simulink model "FieLew95_r2018a"  (R2018a)
settings: Solver=ode1  StartTime=0.0  StopTime=10  FixedStep=0.01  RelTol=1e-5  EnableMultiTasking=on
libraries: simulink x1
settings Model: Creator=dwbertol  LastModifiedBy=dwbertol
settings DataIOCC: LimitDataPoints=on  SaveFormat=Array  SignalLoggingSaveFormat=ModelDataLogs
settings OptimizationCC: ExpressionDepthLimit=2147483647  LifeSpan=inf
settings DebuggingCC: UnderspecifiedInitializationDetection=Classic  MergeDetectMultiDrivingBlocksExec=none  SolverPrmCheckMsg=warning  FcnCallInpInsideContextMsg=warning  StateNameClashWarn=warning  SFUnexpectedBacktrackingDiag=warning  SFNoUnconditionalDefaultTransitionDiag=warning  SFExecutionAtInitializationDiag=none
settings HardwareCC: ProdBitPerPointer=32  ProdBitPerSizeT=32  ProdBitPerPtrDiffT=32  ProdLargestAtomicFloat=None  ProdIntDivRoundTo=Undefined  ProdEndianess=Unspecified  ProdWordSize=32  ProdHWDeviceType=32-bit Generic
settings ModelReferenceCC: PropagateSignalLabelsOutOfModel=off
settings CodeAppCC: StateflowObjectComments=on
settings GRTTargetCC: TargetLangStandard=C89/C90 (ANSI)  GeneratePreprocessorConditionals=Disable all  CombineOutputUpdateFcns=off  GRTInterface=on
settings ConfigComp: CovMetricSettings=dw  CovHtmlReporting=on  CovSaveCumulativeToWorkspaceVar=on  CovSaveSingleToWorkspaceVar=on  CovExternalEMLEnable=off

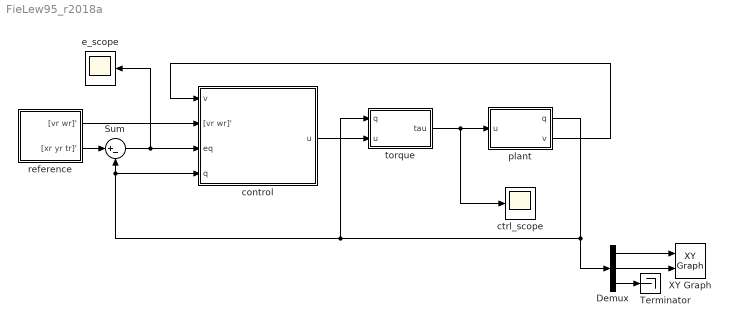
== system FieLew95_r2018a ==
  Demux : Demux  Outputs=3
  Sum : Sum  Inputs=|+-  AccumDataTypeStr=double
  Terminator : Terminator
  XY Graph : simulink/Sinks/XY Graph  xmin=0  xmax=7  ymin=0  ymax=7  st=-1
  control : Subsystem  mask{k1=20, k4=2, am=1, fn=2.4}
      mask prompts: am "Amortecimento"; fn "Frequência Natural"
      mask init:
      | k2 = (fn/0.5)^2;
      | k3 = am*2*(fn/0.5);
  ctrl_scope : Scope
  e_scope : Scope
  plant : Subsystem  mask{u_flag=Torque Rodas (mod. dinâmico), qi=[1 0.8 0]', r=0.05, l=0.3, a=0, b=0, m=10, ir=0.05, irod=0.002}
      mask prompts: u_flag "Entrada de controle"; qi "Postura inicial [x y theta]'"; r "Raio da roda (m)"; l "Distância entre rodas (m)"; a "Deslocamento de P no eixo de simetria"; b "Deslocamento de P no eixo das rodas"; m "Massa do robô (kg)"; ir "Inércia do Robô (Nm)"; irod "Inércia das Rodas (Nm)"
      mask init:
      | q0 = [qi(1) qi(2) qi(3) 0 0];
      mask TypeOptions u_flag: Velocidade Rodas (mod. cinemático) | Velocidade Corpo (mod. cinemático) | Torque Rodas (mod. dinâmico) | Torque Corpo (mod. dinâmico)
  reference : Subsystem  mask{qi=[1 1 (26*pi)/180]', r=0.1953, l=0.393, a=0, b=0}
      mask prompts: qi "Postura inicial [x y theta]'"; r "Raio da roda (m)"; l "Distância entre rodas (m)"; a "Deslocamento de P no eixo de simetria"; b "Deslocamento de P no eixo das rodas"
      mask init:
      | q0 = [qi(1) qi(2) qi(3)];
  torque : Subsystem  mask{r=0.05, l=0.3, a=0, b=0, m=10, ir=0.05, irod=0.002}
      mask prompts: r "Raio da roda (m)"; l "Distância entre rodas (m)"; a "Deslocamento de P no eixo de simetria"; b "Deslocamento de P no eixo das rodas"; m "Massa do robô (kg)"; ir "Inércia do Robô (Nm)"; irod "Inércia das Rodas (Nm)"
  wires:
  plant/1(q) -> Demux/1, Sum/2, control/4(q), torque/1(q)
  reference/2("[xr yr tr]' ") -> Sum/1
  Demux/3 -> Terminator/1
  Demux/2 -> XY Graph/2
  Demux/1 -> XY Graph/1
  Sum/1 -> control/3(eq), e_scope/1
  control/1(u) -> torque/2(u)
  reference/1("[vr wr]' ") -> control/2("[vr wr]'")
  plant/2(v) -> control/1(v)
  torque/1(tau) -> ctrl_scope/1, plant/1(u)

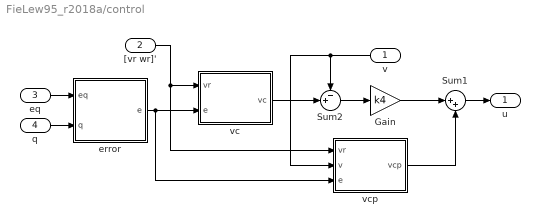
== system FieLew95_r2018a/control ==
  v : Inport
  "[vr wr]'" : Inport  Port=2
  eq : Inport  Port=3
  q : Inport  Port=4
  Gain : Gain  Gain=k4
  Sum1 : Sum  Inputs=|++  AccumDataTypeStr=double
  Sum2 : Sum  Inputs=-+|  AccumDataTypeStr=double
  error : MATLAB Function  TreatAsAtomicUnit=on
  vc : MATLAB Function  TreatAsAtomicUnit=on
  vcp : MATLAB Function  TreatAsAtomicUnit=on
  u : Outport
  wires:
  eq/1 -> error/1(eq)
  Sum1/1 -> u/1
  v/1 -> vcp/2(v), Sum2/1
  q/1 -> error/2(q)
  "[vr wr]'"/1 -> vc/1(vr), vcp/1(vr)
  error/1(e) -> vcp/3(e), vc/2(e)
  vc/1(vc) -> Sum2/2
  Gain/1 -> Sum1/1
  vcp/1(vcp) -> Sum1/2
  Sum2/1 -> Gain/1

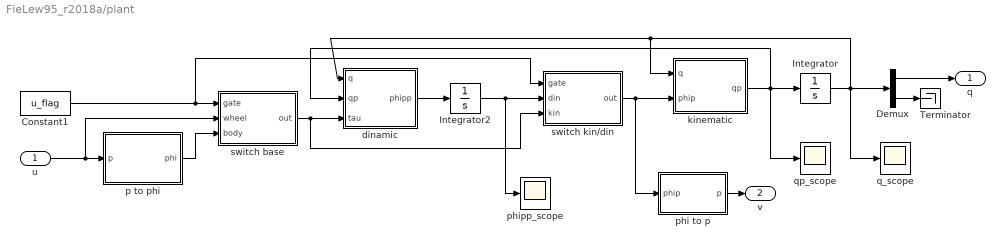
== system FieLew95_r2018a/plant ==
  u : Inport
  Constant1 : Constant  Value=u_flag
  Demux : Demux  Outputs=[3 2]
  Integrator : Integrator  InitialCondition=q0
  Integrator2 : Integrator  InitialCondition=[0 0]'
  Terminator : Terminator
  dinamic : MATLAB Function  TreatAsAtomicUnit=on
  kinematic : MATLAB Function  TreatAsAtomicUnit=on
  p to phi : MATLAB Function  TreatAsAtomicUnit=on
  phi to p : MATLAB Function  TreatAsAtomicUnit=on
  phipp_scope : Scope
  q_scope : Scope
  qp_scope : Scope
  switch base : MATLAB Function  TreatAsAtomicUnit=on
  switch kin/din : MATLAB Function  TreatAsAtomicUnit=on
  q : Outport
  v : Outport  Port=2
  wires:
  switch base/1(out) -> switch kin/din/3(kin), dinamic/3(tau)
  p to phi/1(phi) -> switch base/3(body)
  Constant1/1 -> switch kin/din/1(gate), switch base/1(gate)
  phi to p/1(p) -> v/1
  dinamic/1(phipp) -> Integrator2/1
  Demux/2 -> Terminator/1
  Demux/1 -> q/1
  Integrator/1 -> Demux/1, dinamic/1(q), kinematic/1(q), q_scope/1
  kinematic/1(qp) -> qp_scope/1, Integrator/1, dinamic/2(qp)
  switch kin/din/1(out) -> phi to p/1(phip), kinematic/2(phip)
  Integrator2/1 -> switch kin/din/2(din), phipp_scope/1
  u/1 -> switch base/2(wheel), p to phi/1(p)

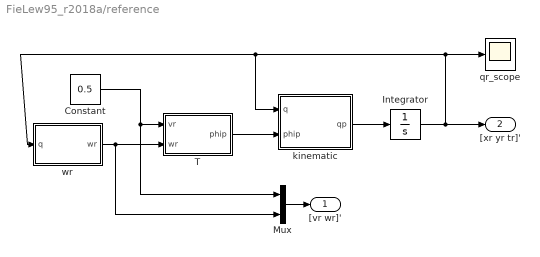
== system FieLew95_r2018a/reference ==
  Constant : Constant  Value=0.5
  Integrator : Integrator  InitialCondition=q0
  Mux : Mux  Inputs=2
  T : MATLAB Function  TreatAsAtomicUnit=on
  kinematic : MATLAB Function  TreatAsAtomicUnit=on
  qr_scope : Scope
  wr : MATLAB Function  TreatAsAtomicUnit=on
  "[vr wr]' " : Outport
  "[xr yr tr]' " : Outport  Port=2
  wires:
  kinematic/1(qp) -> Integrator/1
  T/1(phip) -> kinematic/2(phip)
  Mux/1 -> "[vr wr]' "/1
  wr/1(wr) -> T/2(wr), Mux/2
  Constant/1 -> T/1(vr), Mux/1
  Integrator/1 -> "[xr yr tr]' "/1, wr/1(q), kinematic/1(q), qr_scope/1

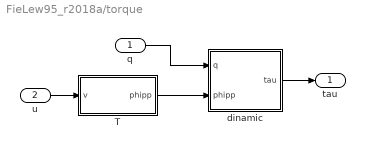
== system FieLew95_r2018a/torque ==
  q : Inport
  u : Inport  Port=2
  T : MATLAB Function  TreatAsAtomicUnit=on
  dinamic : MATLAB Function  TreatAsAtomicUnit=on
  tau : Outport
  wires:
  T/1(phipp) -> dinamic/2(phipp)
  q/1 -> dinamic/1(q)
  u/1 -> T/1(v)
  dinamic/1(tau) -> tau/1

== matlab function FieLew95_r2018a/control/error ==
  data: eq input; e output; q input
function e = fcn(eq,q)
%#eml

 Te = [cos(q(3)) sin(q(3)) 0; -sin(q(3)) cos(q(3)) 0; 0 0 1];
 
 e = Te*eq;

end

== matlab function FieLew95_r2018a/control/vc ==
  data: vr input; e input; vc output; k1 parameter; k2 parameter; k3 parameter
function vc = fcn(vr,e,k1,k2,k3)
%#eml

 vc = [vr(1)*cos(e(3))+k1*e(1);vr(2)+k2*vr(1)*e(2)+k3*vr(1)*sin(e(3))];
 
end

== matlab function FieLew95_r2018a/control/vcp ==
  data: vr input; v input; e input; vcp output; k1 parameter; k2 parameter; k3 parameter
function vcp = fcn(vr,v,e,k1,k2,k3)
%#eml

 ep = [v(2)*e(2)-v(1)+vr(1)*cos(e(3));-v(2)*e(1)+vr(1)*sin(e(3));vr(2)-v(2)];
 vcp = [k1 0 -vr(1)*sin(e(3)); 0 k2*vr(1) k3*vr(1)*cos(e(3))]*ep;
 
end

== matlab function FieLew95_r2018a/plant/dinamic ==
  data: r parameter; l parameter; a parameter; b parameter; m parameter; ir parameter; irod parameter; q input; qp input; tau input; phipp output
function phipp = fcn(r,l,a,b,m,ir,irod,q,qp,tau)
%#eml

 d = l/2;
 c = r/(2*d);
 be = d+b;
 bd = d-b;

 iee = irod;
 idd = irod;
 
 t = q(3);
 %tp = qp(3);
 
 R = [cos(t) sin(t) 0;-sin(t) cos(t) 0;0 0 1];
 %Rp = [-sin(t)*tp cos(t)*tp 0; -cos(t)*tp -sin(t)*tp 0; 0 0 0];

 Sig = [c*be c*bd;c*a -c*a; c -c];

 S = [R'*Sig;eye(2)];
 %Sp = [Rp'*Sig; zeros(2)];

 m1 = m*(a*sin(t)+b*cos(t));
 m2 = m*(a*cos(t)-b*sin(t));

 M = [m 0 m1 0 0;0 m -m2 0 0;m1 -m2 ir 0 0;0 0 0 idd 0;0 0 0 0 iee];

 %C = [0 0 m*(a*cos(t)-b*sin(t))*tp 0 0;...
 %     0 0 m*(a*sin(t)+b*cos(t))*tp 0 0;...
 %     0 0 0 0 0;0 0 0 0 0;0 0 0 0 0];
 
 %N = [0 0;0 0;0 0;1 0;0 1];

 H = S'*M*S;
 %F = S'*M*Sp+S'*C*S;
  
%  vp = -10*qp(4) + 9.5*u(1);
%  wp = -10*qp(5) + 10.5*u(2);

 phipp = H\tau;
end

== matlab function FieLew95_r2018a/reference/T ==
  data: r parameter; l parameter; phip output; vr input; wr input
function phip = fcn(r,l,vr,wr)
%#eml

 d = l/2;

 E = [1/r d/r;1/r -d/r];

 phip = E*[vr wr]';

end

== matlab function FieLew95_r2018a/plant/switch base ==
  data: gate input; wheel input; body input; out output
function out = fcn(gate,wheel,body)
%#eml

 gate = mod(gate,2);
 
 if gate == 0
   out = body;
 else
   out = wheel;
 end
end

== matlab function FieLew95_r2018a/plant/switch kin/din ==
  data: gate input; din input; kin input; out output
function out = fcn(gate,din,kin)
%#eml

 if gate <= 2
   out = kin;
 else
   out = din;
 end
end

== matlab function FieLew95_r2018a/torque/T ==
  data: r parameter; l parameter; v input; phipp output
function phipp = fcn(r,l,v)
%#eml

 d = l/2;

 E = [1/r d/r;1/r -d/r];

 phipp = E*v;

end

== matlab function FieLew95_r2018a/torque/dinamic ==
  data: r parameter; l parameter; a parameter; b parameter; m parameter; ir parameter; irod parameter; q input; phipp input; tau output
function tau = fcn(r,l,a,b,m,ir,irod,q,phipp)
%#eml

 d = l/2;
 c = r/(2*d);
 be = d+b;
 bd = d-b;

 iee = irod;
 idd = irod;
 
 t = q(3);
 
 R = [cos(t) sin(t) 0;-sin(t) cos(t) 0;0 0 1];

 Sig = [c*be c*bd;c*a -c*a; c -c];

 S = [R'*Sig;eye(2)];

 m1 = m*(a*sin(t)+b*cos(t));
 m2 = m*(a*cos(t)-b*sin(t));

 M = [m 0 m1 0 0;0 m -m2 0 0;m1 -m2 ir 0 0;0 0 0 idd 0;0 0 0 0 iee];

 H = S'*M*S;
 
 tau = H*phipp;
end

== matlab function FieLew95_r2018a/reference/wr ==
  data: q input; wr output
function wr = fcn(q)
%#eml

 if q(1) < 3 && q(2) < 2;
   wr = 0;
 else
   wr = 0.125;
 end
 
end

== matlab function FieLew95_r2018a/reference/kinematic ==
  data: r parameter; l parameter; a parameter; b parameter; q input; phip input; qp output
function qp = fcn(r,l,a,b,q,phip)
%#eml

 d = l/2;
 c = r/(2*d);

 t = q(3);
 
 be = d+b;
 bd = d-b;

 S = [c*(be*cos(t)-a*sin(t)) c*(bd*cos(t)+a*sin(t));...
      c*(be*sin(t)+a*cos(t)) c*(bd*sin(t)-a*cos(t));...
      c -c];

 qp = S*phip;

end

== matlab function FieLew95_r2018a/plant/kinematic ==
  data: r parameter; l parameter; a parameter; b parameter; q input; phip input; qp output
function qp = fcn(r,l,a,b,q,phip)
%#eml

 d = l/2;
 c = r/(2*d);

 t = q(3);
 
 be = d+b;
 bd = d-b;

 S = [c*(be*cos(t)-a*sin(t)) c*(bd*cos(t)+a*sin(t));...
      c*(be*sin(t)+a*cos(t)) c*(bd*sin(t)-a*cos(t));...
      c -c;
      1 0;
      0 1];

 qp = S*phip;

end

== matlab function FieLew95_r2018a/plant/p to phi ==
  data: r parameter; l parameter; p input; phi output
function phi = fcn(r,l,p)
%#eml

 d = l/2;

 E = [1/r d/r;1/r -d/r];

 phi = E*p;

end

== matlab function FieLew95_r2018a/plant/phi to p ==
  data: r parameter; l parameter; phip input; p output
function p = fcn(r,l,phip)
%#eml

 d = l/2;

 E = [1/r d/r;1/r -d/r];

 p = E\phip;

end
